simulink library "simetranss"  (R2024b)
settings: Solver=VariableStepAuto  StartTime=0.0  StopTime=10.0  RelTol=1e-3
PostLoadFcn:
  | Ts=1e-6
InitFcn:
  | Ts=1e-6
undefined symbols (not defined in the file): C, C_601, C_603, C_606, CC, Csnu, Csnubber, DiscIntNeverNeededParam, DPL, DPL1ph, FluxTable, ft2km, gcbh, h, Half, Imap2, L, L_601, L_603, L_606, Lbase, LpejoSw, Newton, R_601, R_603, R_606, Raphson, ResistanceM, Roff, Ron, RotorAngles, Rsnu, Rsnubber, Rt4, SampleTime, simetran, sps, sps_rtmsupport, StatorCurrents, T_2wind_ratio, T_Lpu, T_Lpu_pri, T_Rpu, T_Rpu_pri, T_Vpri, T_Vpri_15comp, T_Vsec, Ti, Ts_Power, Z, Zbase, Zm
libraries: fl_lib x248, ee_lib x146, nesl_utility x122, $bdroot x29, simulink x15, eeGeneralControl x2, spsStairGeneratorLib x2, artemis x1
(part 5 of 12)

== system simetranss/Lines/mate_3ph_piline ==
  Capacitor : ee_lib/Passive/Capacitor  cap_option=ee.enum.passive.capacitor.capOption.const  c=C12*len/2 F  Cvec=[1e-05, 1e-06] F  Vvec=[0, 10] V  CV_table_symmetry=ee.enum.passive.capacitor.tableSymmetry.yes  f_vec=[1, 10] kHz  DFext_vec=[.8, 1.2]  enable_C_tol=ee.enum.toleranceApplication.none  averaging_period=0 s  C_tol=5  tol_distribution=ee.enum.toleranceDistribution.uniform  nSigma=4  r=0 Ohm  g=0 1/Ohm  enable_operating_limits=ee.enum.enable.no  operating_limit_action=ee.enum.passive.reportOpLim.warn  max_working_voltage_range=[-25, 25] V  power_rating=1 W  maxTemperature=85 degC  thermalEnable=false  thermalMass=1 J/K  fault_action=simscape.enum.assert.action.none  t_fault=1 s  i_specify=off  i_priority=None  i=0 A  i_nominal_specify=off  i_nominal_value=1  i_nominal_unit=A  v_specify=off  v_priority=None  v=0 V  v_nominal_specify=off  v_nominal_value=1  v_nominal_unit=V  vc_specify=off  vc_priority=High  vc=0 V  vc_nominal_specify=off  vc_nominal_value=1  vc_nominal_unit=V  T_specify=off  T_priority=None  T=298.15 K  T_nominal_specify=off  T_nominal_value=1  T_nominal_unit=K
  Capacitor1 : ee_lib/Passive/Capacitor  cap_option=ee.enum.passive.capacitor.capOption.const  c=C23*len/2 F  Cvec=[1e-05, 1e-06] F  Vvec=[0, 10] V  CV_table_symmetry=ee.enum.passive.capacitor.tableSymmetry.yes  f_vec=[1, 10] kHz  DFext_vec=[.8, 1.2]  enable_C_tol=ee.enum.toleranceApplication.none  averaging_period=0 s  C_tol=5  tol_distribution=ee.enum.toleranceDistribution.uniform  nSigma=4  r=0 Ohm  g=0 1/Ohm  enable_operating_limits=ee.enum.enable.no  operating_limit_action=ee.enum.passive.reportOpLim.warn  max_working_voltage_range=[-25, 25] V  power_rating=1 W  maxTemperature=85 degC  thermalEnable=false  thermalMass=1 J/K  fault_action=simscape.enum.assert.action.none  t_fault=1 s  i_specify=off  i_priority=None  i=0 A  i_nominal_specify=off  i_nominal_value=1  i_nominal_unit=A  v_specify=off  v_priority=None  v=0 V  v_nominal_specify=off  v_nominal_value=1  v_nominal_unit=V  vc_specify=off  vc_priority=High  vc=0 V  vc_nominal_specify=off  vc_nominal_value=1  vc_nominal_unit=V  T_specify=off  T_priority=None  T=298.15 K  T_nominal_specify=off  T_nominal_value=1  T_nominal_unit=K
  Capacitor10 : ee_lib/Passive/Capacitor  cap_option=ee.enum.passive.capacitor.capOption.const  c=C22*len/2 F  Cvec=[1e-05, 1e-06] F  Vvec=[0, 10] V  CV_table_symmetry=ee.enum.passive.capacitor.tableSymmetry.yes  f_vec=[1, 10] kHz  DFext_vec=[.8, 1.2]  enable_C_tol=ee.enum.toleranceApplication.none  averaging_period=0 s  C_tol=5  tol_distribution=ee.enum.toleranceDistribution.uniform  nSigma=4  r=0 Ohm  g=0 1/Ohm  enable_operating_limits=ee.enum.enable.no  operating_limit_action=ee.enum.passive.reportOpLim.warn  max_working_voltage_range=[-25, 25] V  power_rating=1 W  maxTemperature=85 degC  thermalEnable=false  thermalMass=1 J/K  fault_action=simscape.enum.assert.action.none  t_fault=1 s  i_specify=off  i_priority=None  i=0 A  i_nominal_specify=off  i_nominal_value=1  i_nominal_unit=A  v_specify=off  v_priority=None  v=0 V  v_nominal_specify=off  v_nominal_value=1  v_nominal_unit=V  vc_specify=off  vc_priority=High  vc=0 V  vc_nominal_specify=off  vc_nominal_value=1  vc_nominal_unit=V  T_specify=off  T_priority=None  T=298.15 K  T_nominal_specify=off  T_nominal_value=1  T_nominal_unit=K
  Capacitor11 : ee_lib/Passive/Capacitor  cap_option=ee.enum.passive.capacitor.capOption.const  c=C33*len/2 F  Cvec=[1e-05, 1e-06] F  Vvec=[0, 10] V  CV_table_symmetry=ee.enum.passive.capacitor.tableSymmetry.yes  f_vec=[1, 10] kHz  DFext_vec=[.8, 1.2]  enable_C_tol=ee.enum.toleranceApplication.none  averaging_period=0 s  C_tol=5  tol_distribution=ee.enum.toleranceDistribution.uniform  nSigma=4  r=0 Ohm  g=0 1/Ohm  enable_operating_limits=ee.enum.enable.no  operating_limit_action=ee.enum.passive.reportOpLim.warn  max_working_voltage_range=[-25, 25] V  power_rating=1 W  maxTemperature=85 degC  thermalEnable=false  thermalMass=1 J/K  fault_action=simscape.enum.assert.action.none  t_fault=1 s  i_specify=off  i_priority=None  i=0 A  i_nominal_specify=off  i_nominal_value=1  i_nominal_unit=A  v_specify=off  v_priority=None  v=0 V  v_nominal_specify=off  v_nominal_value=1  v_nominal_unit=V  vc_specify=off  vc_priority=High  vc=0 V  vc_nominal_specify=off  vc_nominal_value=1  vc_nominal_unit=V  T_specify=off  T_priority=None  T=298.15 K  T_nominal_specify=off  T_nominal_value=1  T_nominal_unit=K
  Capacitor2 : ee_lib/Passive/Capacitor  cap_option=ee.enum.passive.capacitor.capOption.const  c=C13*len/2 F  Cvec=[1e-05, 1e-06] F  Vvec=[0, 10] V  CV_table_symmetry=ee.enum.passive.capacitor.tableSymmetry.yes  f_vec=[1, 10] kHz  DFext_vec=[.8, 1.2]  enable_C_tol=ee.enum.toleranceApplication.none  averaging_period=0 s  C_tol=5  tol_distribution=ee.enum.toleranceDistribution.uniform  nSigma=4  r=0 Ohm  g=0 1/Ohm  enable_operating_limits=ee.enum.enable.no  operating_limit_action=ee.enum.passive.reportOpLim.warn  max_working_voltage_range=[-25, 25] V  power_rating=1 W  maxTemperature=85 degC  thermalEnable=false  thermalMass=1 J/K  fault_action=simscape.enum.assert.action.none  t_fault=1 s  i_specify=off  i_priority=None  i=0 A  i_nominal_specify=off  i_nominal_value=1  i_nominal_unit=A  v_specify=off  v_priority=None  v=0 V  v_nominal_specify=off  v_nominal_value=1  v_nominal_unit=V  vc_specify=off  vc_priority=High  vc=0 V  vc_nominal_specify=off  vc_nominal_value=1  vc_nominal_unit=V  T_specify=off  T_priority=None  T=298.15 K  T_nominal_specify=off  T_nominal_value=1  T_nominal_unit=K
  Capacitor3 : ee_lib/Passive/Capacitor  cap_option=ee.enum.passive.capacitor.capOption.const  c=C23*len/2 F  Cvec=[1e-05, 1e-06] F  Vvec=[0, 10] V  CV_table_symmetry=ee.enum.passive.capacitor.tableSymmetry.yes  f_vec=[1, 10] kHz  DFext_vec=[.8, 1.2]  enable_C_tol=ee.enum.toleranceApplication.none  averaging_period=0 s  C_tol=5  tol_distribution=ee.enum.toleranceDistribution.uniform  nSigma=4  r=0 Ohm  g=0 1/Ohm  enable_operating_limits=ee.enum.enable.no  operating_limit_action=ee.enum.passive.reportOpLim.warn  max_working_voltage_range=[-25, 25] V  power_rating=1 W  maxTemperature=85 degC  thermalEnable=false  thermalMass=1 J/K  fault_action=simscape.enum.assert.action.none  t_fault=1 s  i_specify=off  i_priority=None  i=0 A  i_nominal_specify=off  i_nominal_value=1  i_nominal_unit=A  v_specify=off  v_priority=None  v=0 V  v_nominal_specify=off  v_nominal_value=1  v_nominal_unit=V  vc_specify=off  vc_priority=High  vc=0 V  vc_nominal_specify=off  vc_nominal_value=1  vc_nominal_unit=V  T_specify=off  T_priority=None  T=298.15 K  T_nominal_specify=off  T_nominal_value=1  T_nominal_unit=K
  Capacitor4 : ee_lib/Passive/Capacitor  cap_option=ee.enum.passive.capacitor.capOption.const  c=C12*len/2 F  Cvec=[1e-05, 1e-06] F  Vvec=[0, 10] V  CV_table_symmetry=ee.enum.passive.capacitor.tableSymmetry.yes  f_vec=[1, 10] kHz  DFext_vec=[.8, 1.2]  enable_C_tol=ee.enum.toleranceApplication.none  averaging_period=0 s  C_tol=5  tol_distribution=ee.enum.toleranceDistribution.uniform  nSigma=4  r=0 Ohm  g=0 1/Ohm  enable_operating_limits=ee.enum.enable.no  operating_limit_action=ee.enum.passive.reportOpLim.warn  max_working_voltage_range=[-25, 25] V  power_rating=1 W  maxTemperature=85 degC  thermalEnable=false  thermalMass=1 J/K  fault_action=simscape.enum.assert.action.none  t_fault=1 s  i_specify=off  i_priority=None  i=0 A  i_nominal_specify=off  i_nominal_value=1  i_nominal_unit=A  v_specify=off  v_priority=None  v=0 V  v_nominal_specify=off  v_nominal_value=1  v_nominal_unit=V  vc_specify=off  vc_priority=High  vc=0 V  vc_nominal_specify=off  vc_nominal_value=1  vc_nominal_unit=V  T_specify=off  T_priority=None  T=298.15 K  T_nominal_specify=off  T_nominal_value=1  T_nominal_unit=K
  Capacitor5 : ee_lib/Passive/Capacitor  cap_option=ee.enum.passive.capacitor.capOption.const  c=C13*len/2 F  Cvec=[1e-05, 1e-06] F  Vvec=[0, 10] V  CV_table_symmetry=ee.enum.passive.capacitor.tableSymmetry.yes  f_vec=[1, 10] kHz  DFext_vec=[.8, 1.2]  enable_C_tol=ee.enum.toleranceApplication.none  averaging_period=0 s  C_tol=5  tol_distribution=ee.enum.toleranceDistribution.uniform  nSigma=4  r=0 Ohm  g=0 1/Ohm  enable_operating_limits=ee.enum.enable.no  operating_limit_action=ee.enum.passive.reportOpLim.warn  max_working_voltage_range=[-25, 25] V  power_rating=1 W  maxTemperature=85 degC  thermalEnable=false  thermalMass=1 J/K  fault_action=simscape.enum.assert.action.none  t_fault=1 s  i_specify=off  i_priority=None  i=0 A  i_nominal_specify=off  i_nominal_value=1  i_nominal_unit=A  v_specify=off  v_priority=None  v=0 V  v_nominal_specify=off  v_nominal_value=1  v_nominal_unit=V  vc_specify=off  vc_priority=High  vc=0 V  vc_nominal_specify=off  vc_nominal_value=1  vc_nominal_unit=V  T_specify=off  T_priority=None  T=298.15 K  T_nominal_specify=off  T_nominal_value=1  T_nominal_unit=K
  Capacitor6 : ee_lib/Passive/Capacitor  cap_option=ee.enum.passive.capacitor.capOption.const  c=C11*len/2 F  Cvec=[1e-05, 1e-06] F  Vvec=[0, 10] V  CV_table_symmetry=ee.enum.passive.capacitor.tableSymmetry.yes  f_vec=[1, 10] kHz  DFext_vec=[.8, 1.2]  enable_C_tol=ee.enum.toleranceApplication.none  averaging_period=0 s  C_tol=5  tol_distribution=ee.enum.toleranceDistribution.uniform  nSigma=4  r=0 Ohm  g=0 1/Ohm  enable_operating_limits=ee.enum.enable.no  operating_limit_action=ee.enum.passive.reportOpLim.warn  max_working_voltage_range=[-25, 25] V  power_rating=1 W  maxTemperature=85 degC  thermalEnable=false  thermalMass=1 J/K  fault_action=simscape.enum.assert.action.none  t_fault=1 s  i_specify=off  i_priority=None  i=0 A  i_nominal_specify=off  i_nominal_value=1  i_nominal_unit=A  v_specify=off  v_priority=None  v=0 V  v_nominal_specify=off  v_nominal_value=1  v_nominal_unit=V  vc_specify=off  vc_priority=High  vc=0 V  vc_nominal_specify=off  vc_nominal_value=1  vc_nominal_unit=V  T_specify=off  T_priority=None  T=298.15 K  T_nominal_specify=off  T_nominal_value=1  T_nominal_unit=K
  Capacitor7 : ee_lib/Passive/Capacitor  cap_option=ee.enum.passive.capacitor.capOption.const  c=C22*len/2 F  Cvec=[1e-05, 1e-06] F  Vvec=[0, 10] V  CV_table_symmetry=ee.enum.passive.capacitor.tableSymmetry.yes  f_vec=[1, 10] kHz  DFext_vec=[.8, 1.2]  enable_C_tol=ee.enum.toleranceApplication.none  averaging_period=0 s  C_tol=5  tol_distribution=ee.enum.toleranceDistribution.uniform  nSigma=4  r=0 Ohm  g=0 1/Ohm  enable_operating_limits=ee.enum.enable.no  operating_limit_action=ee.enum.passive.reportOpLim.warn  max_working_voltage_range=[-25, 25] V  power_rating=1 W  maxTemperature=85 degC  thermalEnable=false  thermalMass=1 J/K  fault_action=simscape.enum.assert.action.none  t_fault=1 s  i_specify=off  i_priority=None  i=0 A  i_nominal_specify=off  i_nominal_value=1  i_nominal_unit=A  v_specify=off  v_priority=None  v=0 V  v_nominal_specify=off  v_nominal_value=1  v_nominal_unit=V  vc_specify=off  vc_priority=High  vc=0 V  vc_nominal_specify=off  vc_nominal_value=1  vc_nominal_unit=V  T_specify=off  T_priority=None  T=298.15 K  T_nominal_specify=off  T_nominal_value=1  T_nominal_unit=K
  Capacitor8 : ee_lib/Passive/Capacitor  cap_option=ee.enum.passive.capacitor.capOption.const  c=C33*len/2 F  Cvec=[1e-05, 1e-06] F  Vvec=[0, 10] V  CV_table_symmetry=ee.enum.passive.capacitor.tableSymmetry.yes  f_vec=[1, 10] kHz  DFext_vec=[.8, 1.2]  enable_C_tol=ee.enum.toleranceApplication.none  averaging_period=0 s  C_tol=5  tol_distribution=ee.enum.toleranceDistribution.uniform  nSigma=4  r=0 Ohm  g=0 1/Ohm  enable_operating_limits=ee.enum.enable.no  operating_limit_action=ee.enum.passive.reportOpLim.warn  max_working_voltage_range=[-25, 25] V  power_rating=1 W  maxTemperature=85 degC  thermalEnable=false  thermalMass=1 J/K  fault_action=simscape.enum.assert.action.none  t_fault=1 s  i_specify=off  i_priority=None  i=0 A  i_nominal_specify=off  i_nominal_value=1  i_nominal_unit=A  v_specify=off  v_priority=None  v=0 V  v_nominal_specify=off  v_nominal_value=1  v_nominal_unit=V  vc_specify=off  vc_priority=High  vc=0 V  vc_nominal_specify=off  vc_nominal_value=1  vc_nominal_unit=V  T_specify=off  T_priority=None  T=298.15 K  T_nominal_specify=off  T_nominal_value=1  T_nominal_unit=K
  Capacitor9 : ee_lib/Passive/Capacitor  cap_option=ee.enum.passive.capacitor.capOption.const  c=C11*len/2 F  Cvec=[1e-05, 1e-06] F  Vvec=[0, 10] V  CV_table_symmetry=ee.enum.passive.capacitor.tableSymmetry.yes  f_vec=[1, 10] kHz  DFext_vec=[.8, 1.2]  enable_C_tol=ee.enum.toleranceApplication.none  averaging_period=0 s  C_tol=5  tol_distribution=ee.enum.toleranceDistribution.uniform  nSigma=4  r=0 Ohm  g=0 1/Ohm  enable_operating_limits=ee.enum.enable.no  operating_limit_action=ee.enum.passive.reportOpLim.warn  max_working_voltage_range=[-25, 25] V  power_rating=1 W  maxTemperature=85 degC  thermalEnable=false  thermalMass=1 J/K  fault_action=simscape.enum.assert.action.none  t_fault=1 s  i_specify=off  i_priority=None  i=0 A  i_nominal_specify=off  i_nominal_value=1  i_nominal_unit=A  v_specify=off  v_priority=None  v=0 V  v_nominal_specify=off  v_nominal_value=1  v_nominal_unit=V  vc_specify=off  vc_priority=High  vc=0 V  vc_nominal_specify=off  vc_nominal_value=1  vc_nominal_unit=V  T_specify=off  T_priority=None  T=298.15 K  T_nominal_specify=off  T_nominal_value=1  T_nominal_unit=K
  Coupled Lines (Three-Phase) : ee_lib/Passive/Lines/Coupled Lines (Three-Phase)  prm=2  La=LL(1,1)*len H  Lb=LL(2,2)*len H  Lc=LL(3,3)*len H  L=1e-3 H  Lmab=LL(1,2)*len H  Lmac=LL(1,3)*len H  Lmbc=LL(2,3)*len H  Lm=3e-4 H  Ra=RR(1,1)*len Ohm  Rb=RR(2,2)*len Ohm  Rc=RR(3,3)*len Ohm  R=0.001 Ohm  Rm=(RR(1,2)+RR(1,3)+RR(2,3))/3*len Ohm  Ga=1e-9 1/Ohm  Gb=1e-9 1/Ohm  Gc=1e-9 1/Ohm  G=1e-9 1/Ohm  I_L_specify=off  I_L_priority=High  I_L=[0, 0, 0] A  I_L_nominal_specify=off  I_L_nominal_value=1  I_L_nominal_unit=A  i_La_specify=off  i_La_priority=High  i_La=0 A  i_La_nominal_specify=off  i_La_nominal_value=1  i_La_nominal_unit=A  i_Lb_specify=off  i_Lb_priority=High  i_Lb=0 A  i_Lb_nominal_specify=off  i_Lb_nominal_value=1  i_Lb_nominal_unit=A  i_Lc_specify=off  i_Lc_priority=High  i_Lc=0 A  i_Lc_nominal_specify=off  i_Lc_nominal_value=1  i_Lc_nominal_unit=A
      settings: InternalSimscapePortConfiguration="{\"Bottom\":[],\"Left\":[{\"id\":\"a1\",\"label\":\"a1\",\"type\":\"foundation.electrical.electrical\"},{\"id\":\"b1\",\"label\":\"b1\",\"type\":\"foundation.electrical.electrical\"},{\"id\":\"c1\",\"label\":\"c1\",\"type\":\"foundation.electrical.electrical\"}],\"Right\":[{\"id\":\"a2\",\"label\":\"a2\",\"type\":\"foundation.electrical.electrical\"},{\"id\":\"b2\",\"label\":\"b2\",\"type\":\"foundation.electrical.electrical\"},{\"id\":\"c2\",\"label\":\"c2\",\"type\":\"foundation.electrical.electrical\"}],\"Top\":[]}"
  Electrical Reference : fl_lib/Electrical/Electrical Elements/Electrical Reference
  Electrical Reference1 : fl_lib/Electrical/Electrical Elements/Electrical Reference
  Phase Splitter1 : ee_lib/Connectors & References/Phase Splitter
  Phase Splitter2 : ee_lib/Connectors & References/Phase Splitter
  abc : PMIOPort  Side=Left
  .abc : PMIOPort  Port=2  Side=Right
  connections:
  .abc/RConn1 -- Phase Splitter1/LConn1
  Phase Splitter2/LConn1 -- abc/RConn1
  Phase Splitter2/RConn3 -- Capacitor1/RConn1 -- Coupled Lines (Three-Phase)/LConn3 -- Capacitor8/LConn1 -- Capacitor2/RConn1
  Coupled Lines (Three-Phase)/RConn3 -- Capacitor3/LConn1 -- Capacitor5/LConn1 -- Phase Splitter1/RConn3 -- Capacitor11/LConn1
  Phase Splitter2/RConn1 -- Capacitor6/LConn1 -- Coupled Lines (Three-Phase)/LConn1 -- Capacitor/LConn1 -- Capacitor2/LConn1
  Phase Splitter1/RConn1 -- Capacitor4/RConn1 -- Capacitor9/LConn1 -- Coupled Lines (Three-Phase)/RConn1 -- Capacitor5/RConn1
  Capacitor7/RConn1 -- Capacitor8/RConn1 -- Capacitor6/RConn1 -- Electrical Reference/LConn1
  Coupled Lines (Three-Phase)/LConn2 -- Capacitor/RConn1 -- Capacitor1/LConn1 -- Phase Splitter2/RConn2 -- Capacitor7/LConn1
  Phase Splitter1/RConn2 -- Capacitor4/LConn1 -- Coupled Lines (Three-Phase)/RConn2 -- Capacitor10/LConn1 -- Capacitor3/RConn1
  Electrical Reference1/LConn1 -- Capacitor9/RConn1 -- Capacitor11/RConn1 -- Capacitor10/RConn1

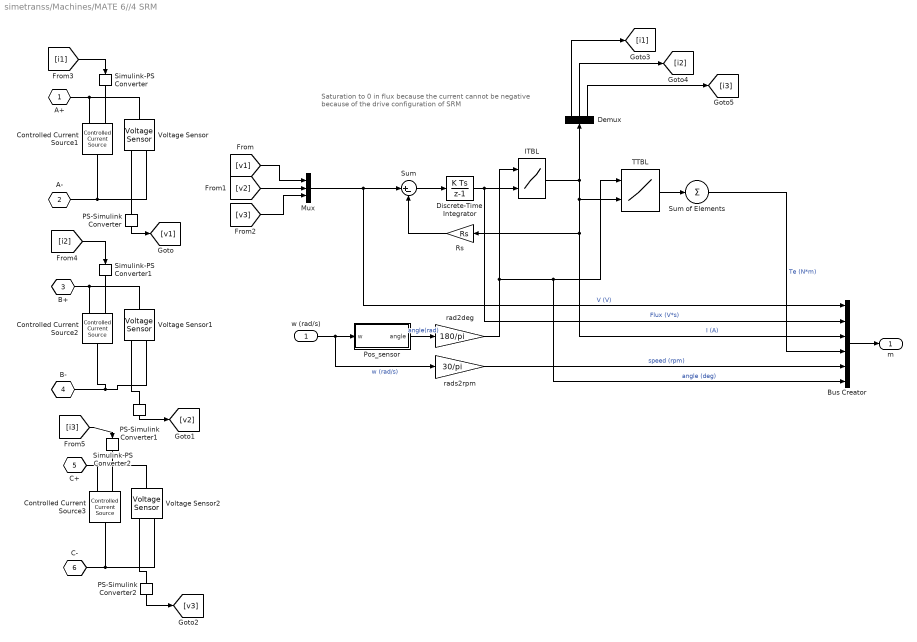
== system simetranss/Machines/MATE 6//4 SRM ==
  note: Saturation to 0 in flux because the current cannot be negative
      | because of the drive configuration of SRM
  w (rad/s) : Inport
  Bus Creator : BusCreator  Inputs=6
  Controlled Current Source1 : fl_lib/Electrical/Electrical Sources/Controlled Current Source
  Controlled Current Source2 : fl_lib/Electrical/Electrical Sources/Controlled Current Source
  Controlled Current Source3 : fl_lib/Electrical/Electrical Sources/Controlled Current Source
  Demux : Demux  Outputs=3
  Discrete-Time Integrator : DiscreteIntegrator  SampleTime=Ts  LimitOutput=on  LowerSaturationLimit=0  ICPrevOutput=DiscIntNeverNeededParam  ICPrevScaledInput=DiscIntNeverNeededParam
  ITBL : Lookup2D  RowIndex=theta2  ColumnIndex=all_flux_value  Table=Imap2'  InputSameDT=off
  Mux : Mux  Inputs=3
  PS-Simulink Converter : nesl_utility/PS-Simulink Converter  PhysicalDomain=network_engine_domain  SubClassName=ps_output  LeftPortType=input  RightPortType=output  PseudoPeriodic=off  Frequencies=[]  VectorFormat=inherit  Unit=inherit  AffineConversion=off
  PS-Simulink Converter1 : nesl_utility/PS-Simulink Converter  PhysicalDomain=network_engine_domain  SubClassName=ps_output  LeftPortType=input  RightPortType=output  PseudoPeriodic=off  Frequencies=[]  VectorFormat=inherit  Unit=inherit  AffineConversion=off
  PS-Simulink Converter2 : nesl_utility/PS-Simulink Converter  PhysicalDomain=network_engine_domain  SubClassName=ps_output  LeftPortType=input  RightPortType=output  PseudoPeriodic=off  Frequencies=[]  VectorFormat=inherit  Unit=inherit  AffineConversion=off
  Pos_sensor : Subsystem
  Rs : Gain  Gain=Rs  SaturateOnIntegerOverflow=on  OutDataTypeStr=Inherit: Same as input  ParamDataTypeStr=Inherit: Same as input
  Simulink-PS Converter : nesl_utility/Simulink-PS Converter  PhysicalDomain=network_engine_domain  SubClassName=ps_input  LeftPortType=input  RightPortType=output  PseudoPeriodic=off  Frequencies=[]  NoiseDistribution=none  NoiseParameters=[]  Unit=1  AffineConversion=off  FilteringAndDerivatives=provide  SimscapeFilterOrder=1  InputFilterTimeConstant=0.001  UdotUserProvided=0
  Simulink-PS Converter1 : nesl_utility/Simulink-PS Converter  PhysicalDomain=network_engine_domain  SubClassName=ps_input  LeftPortType=input  RightPortType=output  PseudoPeriodic=off  Frequencies=[]  NoiseDistribution=none  NoiseParameters=[]  Unit=1  AffineConversion=off  FilteringAndDerivatives=provide  SimscapeFilterOrder=1  InputFilterTimeConstant=0.001  UdotUserProvided=0
  Simulink-PS Converter2 : nesl_utility/Simulink-PS Converter  PhysicalDomain=network_engine_domain  SubClassName=ps_input  LeftPortType=input  RightPortType=output  PseudoPeriodic=off  Frequencies=[]  NoiseDistribution=none  NoiseParameters=[]  Unit=1  AffineConversion=off  FilteringAndDerivatives=provide  SimscapeFilterOrder=1  InputFilterTimeConstant=0.001  UdotUserProvided=0
  Sum : Sum  Inputs=|+-  SaturateOnIntegerOverflow=on
  Sum of Elements : Sum  Inputs=1  SampleTime=Ts
  TTBL : Lookup2D  RowIndex=theta2  ColumnIndex=Icoil2  Table=Temap'  InputSameDT=off
  Voltage Sensor : fl_lib/Electrical/Electrical Sensors/Voltage Sensor
  Voltage Sensor1 : fl_lib/Electrical/Electrical Sensors/Voltage Sensor
  Voltage Sensor2 : fl_lib/Electrical/Electrical Sensors/Voltage Sensor
  rad2deg : Gain  Gain=180/pi  SaturateOnIntegerOverflow=on  OutDataTypeStr=Inherit: Same as input  ParamDataTypeStr=Inherit: Same as input
  rads2rpm : Gain  Gain=30/pi  SaturateOnIntegerOverflow=on  OutDataTypeStr=Inherit: Same as input  ParamDataTypeStr=Inherit: Same as input
  A+ : PMIOPort  Side=Left
  A- : PMIOPort  Port=2  Side=Left
  B+ : PMIOPort  Port=3  Side=Left
  B- : PMIOPort  Port=4  Side=Left
  C+ : PMIOPort  Port=5  Side=Left
  C- : PMIOPort  Port=6  Side=Left
  m : Outport  VectorParamsAs1DForOutWhenUnconnected=off
  wires:
  [i3] -> Simulink-PS Converter2/1
  [i2] -> Simulink-PS Converter1/1
  [i1] -> Simulink-PS Converter/1
  Demux/3 -> [i3]
  Demux/2 -> [i2]
  Demux/1 -> [i1]
  [v3] -> Mux/3
  [v1] -> Mux/1
  [v2] -> Mux/2
  PS-Simulink Converter2/1 -> [v3]
  PS-Simulink Converter1/1 -> [v2]
  PS-Simulink Converter/1 -> [v1]
  rads2rpm/1 -> Bus Creator/5  "speed (rpm)"
  rad2deg/1 -> ITBL/1, Bus Creator/6, TTBL/1  "angle (deg)"
  Pos_sensor/1(angle) -> rad2deg/1  "angle(rad)"
  Mux/1 -> Bus Creator/1, Sum/1  "V (V)"
  Rs/1 -> Sum/2
  Sum of Elements/1 -> Bus Creator/4  "Te (N*m)"
  Bus Creator/1 -> m/1
  w (rad/s)/1 -> Pos_sensor/1(w), rads2rpm/1  "w (rad/s)"
  ITBL/1 -> Demux/1, TTBL/2, Rs/1, Bus Creator/3  "I (A)"
  Sum/1 -> Discrete-Time Integrator/1
  Discrete-Time Integrator/1 -> ITBL/2, Bus Creator/2  "Flux (V*s)"
  TTBL/1 -> Sum of Elements/1
  connections:
  PS-Simulink Converter2/LConn1 -- Voltage Sensor2/RConn1
  Simulink-PS Converter2/RConn1 -- Controlled Current Source3/RConn1
  Controlled Current Source3/RConn2 -- Voltage Sensor2/LConn1 -- C+/RConn1
  Controlled Current Source3/LConn1 -- C-/RConn1 -- Voltage Sensor2/RConn2
  Simulink-PS Converter1/RConn1 -- Controlled Current Source2/RConn1
  PS-Simulink Converter1/LConn1 -- Voltage Sensor1/RConn1
  Controlled Current Source2/RConn2 -- B+/RConn1 -- Voltage Sensor1/LConn1
  Voltage Sensor1/RConn2 -- B-/RConn1 -- Controlled Current Source2/LConn1
  PS-Simulink Converter/LConn1 -- Voltage Sensor/RConn1
  Simulink-PS Converter/RConn1 -- Controlled Current Source1/RConn1
  Voltage Sensor/LConn1 -- A+/RConn1 -- Controlled Current Source1/RConn2
  Controlled Current Source1/LConn1 -- A-/RConn1 -- Voltage Sensor/RConn2

== system simetranss/Machines/MATE Brushless DC Motor (ALT1) ==
  "   w_mec" : Inport
  Bias : Bias  Bias=[0 -2*pi/3 2*pi/3]  SaturateOnIntegerOverflow=off
  Bus Creator : BusCreator  Inputs=5
  Controlled Voltage Source (Three-Phase) : ee_lib/Sources/Controlled Voltage Source (Three-Phase)  input_option=ee.enum.inputType.instantaneous  FRated=60 Hz
      settings: InternalSimscapePortConfiguration="{\"Bottom\":[],\"Left\":[{\"id\":\"S\",\"label\":\"S\",\"type\":\"input\"},{\"id\":\"n\",\"label\":\"n\",\"type\":\"foundation.electrical.electrical\"}],\"Right\":[{\"id\":\"N\",\"label\":\"~\",\"type\":\"foundation.electrical.three_phase\"}],\"Top\":[]}"
  Coupled Lines (Three-Phase) : ee_lib/Passive/Lines/Coupled Lines (Three-Phase)  prm=1  La=1e-3 H  Lb=1e-3 H  Lc=1e-3 H  L=2*Ld H  Lmab=3e-4 H  Lmac=3e-4 H  Lmbc=3e-4 H  Lm=Ld H  Ra=0.001 Ohm  Rb=0.001 Ohm  Rc=0.001 Ohm  R=Rs Ohm  Rm=0 Ohm  Ga=1e-9 1/Ohm  Gb=1e-9 1/Ohm  Gc=1e-9 1/Ohm  G=1e-9 1/Ohm  I_L_specify=off  I_L_priority=High  I_L=[0, 0, 0] A  I_L_nominal_specify=off  I_L_nominal_value=1  I_L_nominal_unit=A  i_La_specify=off  i_La_priority=High  i_La=0 A  i_La_nominal_specify=off  i_La_nominal_value=1  i_La_nominal_unit=A  i_Lb_specify=off  i_Lb_priority=High  i_Lb=0 A  i_Lb_nominal_specify=off  i_Lb_nominal_value=1  i_Lb_nominal_unit=A  i_Lc_specify=off  i_Lc_priority=High  i_Lc=0 A  i_Lc_nominal_specify=off  i_Lc_nominal_value=1  i_Lc_nominal_unit=A
      settings: InternalSimscapePortConfiguration="{\"Bottom\":[],\"Left\":[{\"id\":\"N1\",\"label\":\"~1\",\"type\":\"foundation.electrical.three_phase\"}],\"Right\":[{\"id\":\"N2\",\"label\":\"~2\",\"type\":\"foundation.electrical.three_phase\"}],\"Top\":[]}"
  Current Sensor (Three-Phase) : ee_lib/Sensors & Transducers/Current Sensor (Three-Phase)
  Discrete-Time Integrator : DiscreteIntegrator  InitialCondition=pp*AngInit/180*pi  SampleTime=Ts  ICPrevOutput=DiscIntNeverNeededParam  ICPrevScaledInput=DiscIntNeverNeededParam
  Gain1 : Gain  Gain=1/pp
  Gain3 : Gain  Gain=pp  SaturateOnIntegerOverflow=on  OutDataTypeStr=Inherit: Same as input  ParamDataTypeStr=Inherit: Same as input
  Gain4 : Gain  Gain=-Mf
  PS-Simulink Converter4 : nesl_utility/PS-Simulink Converter  PhysicalDomain=network_engine_domain  SubClassName=ps_output  LeftPortType=input  RightPortType=output  PseudoPeriodic=off  Frequencies=[]  VectorFormat=inherit  Unit=inherit  AffineConversion=off
  Product6 : Product  RndMeth=Zero
  Product8 : Product  SaturateOnIntegerOverflow=on  OutDataTypeStr=Inherit: Same as first input
  Signal Specification : SignalSpecification  Dimensions=3
  Simulink-PS Converter3 : nesl_utility/Simulink-PS Converter  PhysicalDomain=network_engine_domain  SubClassName=ps_input  LeftPortType=input  RightPortType=output  PseudoPeriodic=off  Frequencies=[]  NoiseDistribution=none  NoiseParameters=[]  Unit=1  AffineConversion=off  FilteringAndDerivatives=provide  SimscapeFilterOrder=1  InputFilterTimeConstant=0.001  UdotUserProvided=0
  Sum2 : Sum  Inputs=+  SaturateOnIntegerOverflow=on
  Trigonometric Function1 : Trigonometry
  pole pair1 : Gain  Gain=pp
  "   abc" : PMIOPort  Side=Left
  meas : Outport  VectorParamsAs1DForOutWhenUnconnected=off
  wires:
  [Te] -> Bus Creator/3  "Electric torque (Nm)"
  Bus Creator/1 -> meas/1
  "   w_mec"/1 -> pole pair1/1, [W_m]
  pole pair1/1 -> Discrete-Time Integrator/1, [w_e]  "w_elect"
  Discrete-Time Integrator/1 -> [theta_e], Gain1/1  "theta_elect (rad)"
  [iabc_bldc] -> Signal Specification/1  "Iabc(A)"
  [backemf] -> Bus Creator/2  "Back-EMF (V)"
  Gain1/1 -> [Theta_m]
  [W_m] -> Bus Creator/5  "mec speed (rad_s)"
  [Theta_m] -> Bus Creator/4  "mec angle (rad)"
  [theta_e] -> Bias/1
  Bias/1 -> Trigonometric Function1/1
  [w_e] -> Product6/2
  Trigonometric Function1/1 -> Gain4/1
  Product6/1 -> Simulink-PS Converter3/1, [backemf]  "BackEMF on q axis"
  Gain3/1 -> [Te]
  Product8/1 -> Sum2/1
  [iabc_bldc] -> Product8/2
  [X] -> Product8/1
  Sum2/1 -> Gain3/1
  PS-Simulink Converter4/1 -> [iabc_bldc]
  Gain4/1 -> Product6/1, [X]
  Signal Specification/1 -> Bus Creator/1  "Iabc(A)"
  connections:
  Controlled Voltage Source (Three-Phase)/RConn1 -- Coupled Lines (Three-Phase)/RConn1
  Simulink-PS Converter3/RConn1 -- Controlled Voltage Source (Three-Phase)/LConn1
  PS-Simulink Converter4/LConn1 -- Current Sensor (Three-Phase)/RConn1
  Current Sensor (Three-Phase)/LConn1 -- "   abc"/RConn1
  Coupled Lines (Three-Phase)/LConn1 -- Current Sensor (Three-Phase)/RConn2

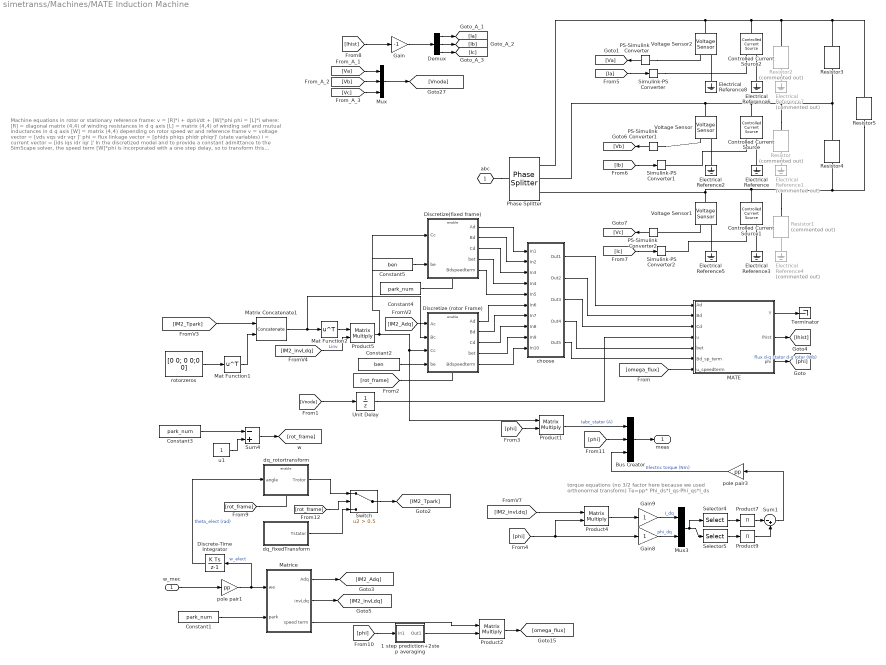
== system simetranss/Machines/MATE Induction Machine ==
  note: Machine equations in rotor or stationary reference frame:
      |
      |   v = [R]*i + dphi/dt + [W]*phi
      | phi = [L]*i
      |
      | where:
      | [R] = diagonal matrix (4,4) of winding resistances in d q axis
      | [L] = matrix (4,4) of winding self and mutual inductances in d q axis
      | [W] = matrix (4,4) depending on rotor speed wr and reference frame
      |
      |   v = voltage vector      = [vds   vqs   vdr   vqr  ]'
      | phi = flux linkage vector = [phids phiqs phidr phiqr]' (state variables)
      |   i = current vector      = [ids   iqs   idr   iqr  ]'
      |
      | In the discretized model and to provide a constant admittance to the SimScape solver, the speed term [W]*phi is incorporated with a one step delay, so to transform this component into an input to the state equations
  note: torque equations
      | (no 3/2 factor here because we used orthonormal transform)
      | Te=pp* Phi_ds*I_qs-Phi_qs*I_ds
  "   w_mec" : Inport
  1 step prediction+2step averaging : Subsystem
  Bus Creator : BusCreator  Inputs=3
  Constant1 : Constant  Value=park_num
  Constant2 : Constant  Value=ben
  Constant3 : Constant  Value=park_num
  Constant4 : Constant  Value=park_num
  Constant5 : Constant  Value=ben
  Controlled Current Source : fl_lib/Electrical/Electrical Sources/Controlled Current Source
  Controlled Current Source1 : fl_lib/Electrical/Electrical Sources/Controlled Current Source
  Controlled Current Source2 : fl_lib/Electrical/Electrical Sources/Controlled Current Source
  Demux : Demux  Outputs=3
      settings: DisplayOption=none
  Discrete-Time Integrator : DiscreteIntegrator  SampleTime=Ts  ICPrevOutput=DiscIntNeverNeededParam  ICPrevScaledInput=DiscIntNeverNeededParam
  Discretize (rotor Frame) : Subsystem
  Discretize(fixed frame) : Subsystem
  Electrical Reference{,2..3,5..6,8} (6 alike) : fl_lib/Electrical/Electrical Elements/Electrical Reference
  Electrical Reference1 : fl_lib/Electrical/Electrical Elements/Electrical Reference  Commented=on
  Electrical Reference4 : fl_lib/Electrical/Electrical Elements/Electrical Reference  Commented=on
  Electrical Reference7 : fl_lib/Electrical/Electrical Elements/Electrical Reference  Commented=on
  Gain : Gain  Gain=-1
  Gain8 : Gain
  Gain9 : Gain
  MATE : Subsystem
  Mat Function1 : Math  Operator=transpose  SignedPower=on
  Mat Function2 : Math  Operator=transpose  SignedPower=on
  Matrice : Subsystem
  Matrix Concatenate1 : Concatenate  Mode=Multidimensional array
  Mux : Mux  Inputs=3
  Mux3 : Mux  Inputs=2
  PS-Simulink Converter : nesl_utility/PS-Simulink Converter  PhysicalDomain=network_engine_domain  SubClassName=ps_output  LeftPortType=input  RightPortType=output  PseudoPeriodic=off  Frequencies=[]  VectorFormat=inherit  Unit=inherit  AffineConversion=off
  PS-Simulink Converter1 : nesl_utility/PS-Simulink Converter  PhysicalDomain=network_engine_domain  SubClassName=ps_output  LeftPortType=input  RightPortType=output  PseudoPeriodic=off  Frequencies=[]  VectorFormat=inherit  Unit=inherit  AffineConversion=off
  PS-Simulink Converter2 : nesl_utility/PS-Simulink Converter  PhysicalDomain=network_engine_domain  SubClassName=ps_output  LeftPortType=input  RightPortType=output  PseudoPeriodic=off  Frequencies=[]  VectorFormat=inherit  Unit=inherit  AffineConversion=off
  Phase Splitter : ee_lib/Connectors & References/Phase Splitter
  Product{1..2,4..5} (4 alike) : Product  Multiplication=Matrix(*)  SaturateOnIntegerOverflow=on  OutDataTypeStr=Inherit: Same as first input
  Product7 : Product  Inputs=1  InputSameDT=on  SaturateOnIntegerOverflow=on  OutDataTypeStr=Inherit: Same as first input
  Product9 : Product  Inputs=1  InputSameDT=on  SaturateOnIntegerOverflow=on  OutDataTypeStr=Inherit: Same as first input
  Resistor : fl_lib/Electrical/Electrical Elements/Resistor  Commented=on  R=ResistanceM(2,2) Ohm  i_specify=off  i_priority=None  i=0 A  i_nominal_specify=off  i_nominal_value=1  i_nominal_unit=A  v_specify=off  v_priority=None  v=0 V  v_nominal_specify=off  v_nominal_value=1  v_nominal_unit=V
  Resistor1 : fl_lib/Electrical/Electrical Elements/Resistor  Commented=on  R=ResistanceM(3,3) Ohm  i_specify=off  i_priority=None  i=0 A  i_nominal_specify=off  i_nominal_value=1  i_nominal_unit=A  v_specify=off  v_priority=None  v=0 V  v_nominal_specify=off  v_nominal_value=1  v_nominal_unit=V
  Resistor2 : fl_lib/Electrical/Electrical Elements/Resistor  Commented=on  R=ResistanceM(1,1) Ohm  i_specify=off  i_priority=None  i=0 A  i_nominal_specify=off  i_nominal_value=1  i_nominal_unit=A  v_specify=off  v_priority=None  v=0 V  v_nominal_specify=off  v_nominal_value=1  v_nominal_unit=V
  Resistor3 : fl_lib/Electrical/Electrical Elements/Resistor  R=ResistanceM(1,2) Ohm  i_specify=off  i_priority=None  i=0 A  i_nominal_specify=off  i_nominal_value=1  i_nominal_unit=A  v_specify=off  v_priority=None  v=0 V  v_nominal_specify=off  v_nominal_value=1  v_nominal_unit=V
  Resistor4 : fl_lib/Electrical/Electrical Elements/Resistor  R=ResistanceM(2,3) Ohm  i_specify=off  i_priority=None  i=0 A  i_nominal_specify=off  i_nominal_value=1  i_nominal_unit=A  v_specify=off  v_priority=None  v=0 V  v_nominal_specify=off  v_nominal_value=1  v_nominal_unit=V
  Resistor5 : fl_lib/Electrical/Electrical Elements/Resistor  R=ResistanceM(1,3) Ohm  i_specify=off  i_priority=None  i=0 A  i_nominal_specify=off  i_nominal_value=1  i_nominal_unit=A  v_specify=off  v_priority=None  v=0 V  v_nominal_specify=off  v_nominal_value=1  v_nominal_unit=V
  Selector4 : Selector  InputPortWidth=8  IndexOptions=Index vector (dialog)  Indices=[1 6]  OutputSizes=1
  Selector5 : Selector  InputPortWidth=8  IndexOptions=Index vector (dialog)  Indices=[2 5]  OutputSizes=1
  Simulink-PS Converter : nesl_utility/Simulink-PS Converter  PhysicalDomain=network_engine_domain  SubClassName=ps_input  LeftPortType=input  RightPortType=output  PseudoPeriodic=off  Frequencies=[]  NoiseDistribution=none  NoiseParameters=[]  Unit=1  AffineConversion=off  FilteringAndDerivatives=provide  SimscapeFilterOrder=1  InputFilterTimeConstant=0.001  UdotUserProvided=0
  Simulink-PS Converter1 : nesl_utility/Simulink-PS Converter  PhysicalDomain=network_engine_domain  SubClassName=ps_input  LeftPortType=input  RightPortType=output  PseudoPeriodic=off  Frequencies=[]  NoiseDistribution=none  NoiseParameters=[]  Unit=1  AffineConversion=off  FilteringAndDerivatives=provide  SimscapeFilterOrder=1  InputFilterTimeConstant=0.001  UdotUserProvided=0
  Simulink-PS Converter2 : nesl_utility/Simulink-PS Converter  PhysicalDomain=network_engine_domain  SubClassName=ps_input  LeftPortType=input  RightPortType=output  PseudoPeriodic=off  Frequencies=[]  NoiseDistribution=none  NoiseParameters=[]  Unit=1  AffineConversion=off  FilteringAndDerivatives=provide  SimscapeFilterOrder=1  InputFilterTimeConstant=0.001  UdotUserProvided=0
  Sum1 : Sum  Inputs=|-+  InputSameDT=on  SaturateOnIntegerOverflow=on  OutDataTypeStr=Inherit: Same as first input
  Sum4 : Sum  Inputs=-+  SaturateOnIntegerOverflow=on
  Switch : Switch  Criteria=u2 > Threshold  Threshold=0.5  SaturateOnIntegerOverflow=off  InputSameDT=off
  Terminator : Terminator
  Unit Delay : UnitDelay  SampleTime=Ts  HasFrameUpgradeWarning=on
  Voltage Sensor : fl_lib/Electrical/Electrical Sensors/Voltage Sensor
  Voltage Sensor1 : fl_lib/Electrical/Electrical Sensors/Voltage Sensor
  Voltage Sensor2 : fl_lib/Electrical/Electrical Sensors/Voltage Sensor
  choose : Subsystem
  dq_fixedTransform : Subsystem
  dq_rotortransform : Subsystem
  pole pair1 : Gain  Gain=pp
  pole pair3 : Gain  Gain=pp
  rotorzeros : Constant  Value=[0 0; 0 0;0 0]
  u1 : Constant
  "   abc" : PMIOPort  Side=Left
  meas : Outport  VectorParamsAs1DForOutWhenUnconnected=off
  wires:
  dq_fixedTransform/1(Tstator) -> Switch/3
  [rot_frame] -> dq_rotortransform/Enable
  [rot_frame] -> Switch/2
  choose/5(Out5) -> MATE/6(Bd_sp_term)
  choose/4(Out4) -> MATE/5(bet)
  choose/3(Out3) -> MATE/3(Cd)
  choose/2(Out2) -> MATE/2(Bd)
  choose/1(Out1) -> MATE/1(Ad)
  Discretize (rotor Frame)/5(Bdspeedterm) -> choose/10(In10)
  Discretize (rotor Frame)/4(bet) -> choose/9(In9)
  Discretize (rotor Frame)/3(Cd) -> choose/8(In8)
  Discretize (rotor Frame)/2(Bd) -> choose/7(In7)
  Discretize (rotor Frame)/1(Ad) -> choose/6(In6)
  Discretize(fixed frame)/5(Bdspeedterm) -> choose/5(In5)
  Discretize(fixed frame)/4(bet) -> choose/4(In4)
  Discretize(fixed frame)/3(Cd) -> choose/3(In3)
  Discretize(fixed frame)/2(Bd) -> choose/2(In2)
  Discretize(fixed frame)/1(Ad) -> choose/1(In1)
  Constant5/1 -> Discretize(fixed frame)/2(be)
  Constant4/1 -> Discretize(fixed frame)/Enable
  [phi] -> Bus Creator/2
  Constant3/1 -> Sum4/1
  u1/1 -> Sum4/2
  [rot_frame] -> Discretize (rotor Frame)/Enable
  Sum4/1 -> [rot_frame]
  [Ic] -> Simulink-PS Converter2/1
  [Ib] -> Simulink-PS Converter1/1
  [Ia] -> Simulink-PS Converter/1
  PS-Simulink Converter2/1 -> [Vc]
  PS-Simulink Converter1/1 -> [Vb]
  PS-Simulink Converter/1 -> [Va]
  Mux/1 -> [Vnode]
  Demux/3 -> [Ic]
  Demux/2 -> [Ib]
  Demux/1 -> [Ia]
  [Vb] -> Mux/2
  [Vc] -> Mux/3
  [Ihist] -> Gain/1
  Gain/1 -> Demux/1
  [Va] -> Mux/1
  Product2/1 -> [omega_flux]
  [phi] -> 1 step prediction+2step averaging/1(In1)
  [omega_flux] -> MATE/7(u_speedterm)
  Mat Function2/1 -> Product5/1
  Constant2/1 -> Discretize (rotor Frame)/4(be)
  [Vnode] -> Unit Delay/1
  [IM2_Tpark] -> Matrix Concatenate1/1
  Mat Function1/1 -> Matrix Concatenate1/2
  rotorzeros/1 -> Mat Function1/1
  Product5/1 -> Discretize (rotor Frame)/3(Cc), Product1/1, Discretize(fixed frame)/1(Cc)
  [IM2_invLdq] -> Product5/2  "Linv"
  Unit Delay/1 -> MATE/4(u)
  Bus Creator/1 -> meas/1
  MATE/3(phi) -> [phi]  "flux d-q stator d-q rotor (Wb)"
  Product1/1 -> Bus Creator/1  "Iabc_stator (A)"
  Matrix Concatenate1/1 -> Discretize (rotor Frame)/2(Bc), Mat Function2/1
  [IM2_Adq] -> Discretize (rotor Frame)/1(Ac)
  [IM2_invLdq] -> Product4/1
  Product4/1 -> Gain9/1
  Gain9/1 -> Mux3/1  "I_dq"
  Gain8/1 -> Mux3/2  "phi_dq"
  Mux3/1 -> Selector5/1, Selector4/1
  Product7/1 -> Sum1/1
  Product9/1 -> Sum1/2
  Selector5/1 -> Product9/1
  Selector4/1 -> Product7/1
  Sum1/1 -> pole pair3/1
  pole pair3/1 -> Bus Creator/3  "Electric torque (Nm)"
  MATE/1(Y) -> Terminator/1
  MATE/2(Ihist) -> [Ihist]
  1 step prediction+2step averaging/1(Out1) -> Product2/2
  [phi] -> Product4/2, Gain8/1
  [phi] -> Product1/2
  Discrete-Time Integrator/1 -> dq_rotortransform/1(angle)  "theta_elect (rad)"
  Matrice/1(Adq) -> [IM2_Adq]
  Matrice/2(invLdq) -> [IM2_invLdq]
  "   w_mec"/1 -> pole pair1/1
  pole pair1/1 -> Discrete-Time Integrator/1, Matrice/1(we)  "w_elect"
  Matrice/3(speed term) -> Product2/1
  Constant1/1 -> Matrice/2(park)
  dq_rotortransform/1(Trotor) -> Switch/1
  Switch/1 -> [IM2_Tpark]
  connections:
  Controlled Current Source1/RConn1 -- Simulink-PS Converter2/RConn1
  Controlled Current Source/RConn1 -- Simulink-PS Converter1/RConn1
  Simulink-PS Converter/RConn1 -- Controlled Current Source2/RConn1
  Voltage Sensor1/RConn1 -- PS-Simulink Converter2/LConn1
  PS-Simulink Converter1/LConn1 -- Voltage Sensor/RConn1
  PS-Simulink Converter/LConn1 -- Voltage Sensor2/RConn1
  Electrical Reference7/LConn1 -- Resistor2/RConn1
  Electrical Reference6/LConn1 -- Controlled Current Source2/RConn2
  Electrical Reference8/LConn1 -- Voltage Sensor2/RConn2
  Phase Splitter/RConn1 -- Voltage Sensor2/LConn1 -- Resistor2/LConn1 -- Resistor3/LConn1 -- Resistor5/LConn1 -- Controlled Current Source2/LConn1
  Electrical Reference4/LConn1 -- Resistor1/RConn1
  Electrical Reference3/LConn1 -- Controlled Current Source1/RConn2
  Electrical Reference5/LConn1 -- Voltage Sensor1/RConn2
  Resistor1/LConn1 -- Resistor4/RConn1 -- Resistor5/RConn1 -- Phase Splitter/RConn3 -- Voltage Sensor1/LConn1 -- Controlled Current Source1/LConn1
  Electrical Reference2/LConn1 -- Voltage Sensor/RConn2
  Electrical Reference1/LConn1 -- Resistor/RConn1
  Resistor/LConn1 -- Resistor3/RConn1 -- Resistor4/LConn1 -- Phase Splitter/RConn2 -- Voltage Sensor/LConn1 -- Controlled Current Source/LConn1
  Electrical Reference/LConn1 -- Controlled Current Source/RConn2
  "   abc"/RConn1 -- Phase Splitter/LConn1

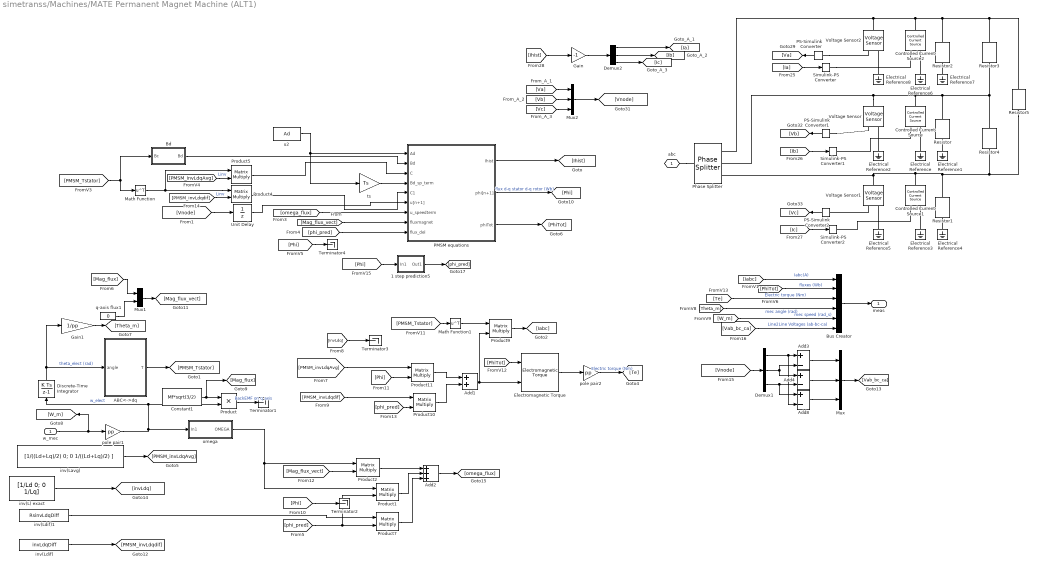
== system simetranss/Machines/MATE Permanent Magnet Machine (ALT1) ==
  "   w_mec" : Inport
  1 step prediction5 : Subsystem
  ABC<->dq : Subsystem
  Add1 : Sum
  Add2 : Sum  Inputs=+++
  Add3 : Sum  Inputs=+-
  Add4 : Sum  Inputs=+-
  Add8 : Sum  Inputs=+-
  Bd : Subsystem
  Bus Creator : BusCreator  Inputs=6
  Constant1 : Constant  Value=Mf*sqrt(3/2)
  Controlled Current Source : fl_lib/Electrical/Electrical Sources/Controlled Current Source
  Controlled Current Source1 : fl_lib/Electrical/Electrical Sources/Controlled Current Source
  Controlled Current Source2 : fl_lib/Electrical/Electrical Sources/Controlled Current Source
  Demux1 : Demux  Outputs=[1 1 1]
  Demux2 : Demux  Outputs=3
      settings: DisplayOption=none
  Discrete-Time Integrator : DiscreteIntegrator  InitialCondition=pp*AngInit/180*pi  SampleTime=Ts  ICPrevOutput=DiscIntNeverNeededParam  ICPrevScaledInput=DiscIntNeverNeededParam
  Electrical Reference{,1..8} (9 alike) : fl_lib/Electrical/Electrical Elements/Electrical Reference
  Electromagnetic Torque : artemis/SSN/SSN rotating machines/SSN Synchronous Machine/Electromagnetic Torque  SystemSampleTime=-1  VariantActivationTime=update diagram  AllowFlexibleInterface=on  Latency=0  AutoFrameSizeCalculation=off
      settings: SourceProductName=Artemis
  Gain : Gain  Gain=-1
  Gain1 : Gain  Gain=1/pp
  Math Function : Math  Operator=transpose  SignedPower=on
  Math Function1 : Math  Operator=transpose  SignedPower=on
  Mux : Mux  Inputs=3
  Mux1 : Mux  Inputs=2
  Mux2 : Mux  Inputs=3
  PMSM equations : Subsystem
  PS-Simulink Converter : nesl_utility/PS-Simulink Converter  PhysicalDomain=network_engine_domain  SubClassName=ps_output  LeftPortType=input  RightPortType=output  PseudoPeriodic=off  Frequencies=[]  VectorFormat=inherit  Unit=inherit  AffineConversion=off
  PS-Simulink Converter1 : nesl_utility/PS-Simulink Converter  PhysicalDomain=network_engine_domain  SubClassName=ps_output  LeftPortType=input  RightPortType=output  PseudoPeriodic=off  Frequencies=[]  VectorFormat=inherit  Unit=inherit  AffineConversion=off
  PS-Simulink Converter2 : nesl_utility/PS-Simulink Converter  PhysicalDomain=network_engine_domain  SubClassName=ps_output  LeftPortType=input  RightPortType=output  PseudoPeriodic=off  Frequencies=[]  VectorFormat=inherit  Unit=inherit  AffineConversion=off
  Phase Splitter : ee_lib/Connectors & References/Phase Splitter
  Product : Product  RndMeth=Zero
  Product{1..2,4..5,7,9..11} (8 alike) : Product  Multiplication=Matrix(*)  SaturateOnIntegerOverflow=on  OutDataTypeStr=Inherit: Same as first input
  Resistor : fl_lib/Electrical/Electrical Elements/Resistor  R=ResistanceM(2,2) Ohm  i_specify=off  i_priority=None  i=0 A  i_nominal_specify=off  i_nominal_value=1  i_nominal_unit=A  v_specify=off  v_priority=None  v=0 V  v_nominal_specify=off  v_nominal_value=1  v_nominal_unit=V
  Resistor1 : fl_lib/Electrical/Electrical Elements/Resistor  R=ResistanceM(3,3) Ohm  i_specify=off  i_priority=None  i=0 A  i_nominal_specify=off  i_nominal_value=1  i_nominal_unit=A  v_specify=off  v_priority=None  v=0 V  v_nominal_specify=off  v_nominal_value=1  v_nominal_unit=V
  Resistor2 : fl_lib/Electrical/Electrical Elements/Resistor  R=ResistanceM(1,1) Ohm  i_specify=off  i_priority=None  i=0 A  i_nominal_specify=off  i_nominal_value=1  i_nominal_unit=A  v_specify=off  v_priority=None  v=0 V  v_nominal_specify=off  v_nominal_value=1  v_nominal_unit=V
  Resistor3 : fl_lib/Electrical/Electrical Elements/Resistor  R=ResistanceM(1,2) Ohm  i_specify=off  i_priority=None  i=0 A  i_nominal_specify=off  i_nominal_value=1  i_nominal_unit=A  v_specify=off  v_priority=None  v=0 V  v_nominal_specify=off  v_nominal_value=1  v_nominal_unit=V
  Resistor4 : fl_lib/Electrical/Electrical Elements/Resistor  R=ResistanceM(2,3) Ohm  i_specify=off  i_priority=None  i=0 A  i_nominal_specify=off  i_nominal_value=1  i_nominal_unit=A  v_specify=off  v_priority=None  v=0 V  v_nominal_specify=off  v_nominal_value=1  v_nominal_unit=V
  Resistor5 : fl_lib/Electrical/Electrical Elements/Resistor  R=ResistanceM(1,3) Ohm  i_specify=off  i_priority=None  i=0 A  i_nominal_specify=off  i_nominal_value=1  i_nominal_unit=A  v_specify=off  v_priority=None  v=0 V  v_nominal_specify=off  v_nominal_value=1  v_nominal_unit=V
  Simulink-PS Converter : nesl_utility/Simulink-PS Converter  PhysicalDomain=network_engine_domain  SubClassName=ps_input  LeftPortType=input  RightPortType=output  PseudoPeriodic=off  Frequencies=[]  NoiseDistribution=none  NoiseParameters=[]  Unit=1  AffineConversion=off  FilteringAndDerivatives=provide  SimscapeFilterOrder=1  InputFilterTimeConstant=0.001  UdotUserProvided=0
  Simulink-PS Converter1 : nesl_utility/Simulink-PS Converter  PhysicalDomain=network_engine_domain  SubClassName=ps_input  LeftPortType=input  RightPortType=output  PseudoPeriodic=off  Frequencies=[]  NoiseDistribution=none  NoiseParameters=[]  Unit=1  AffineConversion=off  FilteringAndDerivatives=provide  SimscapeFilterOrder=1  InputFilterTimeConstant=0.001  UdotUserProvided=0
  Simulink-PS Converter2 : nesl_utility/Simulink-PS Converter  PhysicalDomain=network_engine_domain  SubClassName=ps_input  LeftPortType=input  RightPortType=output  PseudoPeriodic=off  Frequencies=[]  NoiseDistribution=none  NoiseParameters=[]  Unit=1  AffineConversion=off  FilteringAndDerivatives=provide  SimscapeFilterOrder=1  InputFilterTimeConstant=0.001  UdotUserProvided=0
  Terminator{1..4} (4 alike) : Terminator
  Unit Delay : UnitDelay  SampleTime=Ts  HasFrameUpgradeWarning=on
  Voltage Sensor : fl_lib/Electrical/Electrical Sensors/Voltage Sensor
  Voltage Sensor1 : fl_lib/Electrical/Electrical Sensors/Voltage Sensor
  Voltage Sensor2 : fl_lib/Electrical/Electrical Sensors/Voltage Sensor
  inv(L) exact : Constant  Value=[1/Ld 0; 0 1/Lq]
  inv(Lavg) : Constant  Value=[1/((Ld+Lq)/2) 0; 0 1/((Ld+Lq)/2) ]
  inv(Ldif) : Constant  Value=invLdqDiff
  inv(Ldif)1 : Constant  Value=RsinvLdqDiff
  omega : Subsystem
  pole pair1 : Gain  Gain=pp
  pole pair2 : Gain  Gain=pp
  q-axis flux1 : Constant  Value=0
  ts : Gain  Gain=Ts  SaturateOnIntegerOverflow=on  OutDataTypeStr=Inherit: Same as input  ParamDataTypeStr=Inherit: Same as input
  u2 : Constant  Value=Ad
  "   abc" : PMIOPort  Side=Left
  meas : Outport  VectorParamsAs1DForOutWhenUnconnected=off
  wires:
  omega/1(OMEGA) -> Product2/1, Product1/1
  ts/1 -> PMSM equations/4(Bd_sp_term)
  u2/1 -> PMSM equations/1(Ad), ts/1
  [Ihist] -> Gain/1
  Demux2/3 -> [Ic]
  [Ib] -> Simulink-PS Converter1/1
  PS-Simulink Converter/1 -> [Va]
  [Ic] -> Simulink-PS Converter2/1
  PS-Simulink Converter1/1 -> [Vb]
  Demux2/2 -> [Ib]
  [Va] -> Mux2/1
  PS-Simulink Converter2/1 -> [Vc]
  [Vb] -> Mux2/2
  [Ia] -> Simulink-PS Converter/1
  Mux2/1 -> [Vnode]
  Gain/1 -> Demux2/1
  [Vc] -> Mux2/3
  Demux2/1 -> [Ia]
  [Vab_bc_ca] -> Bus Creator/6  "Line2Line Voltages (ab-bc-ca)"
  [Vnode] -> Demux1/1
  Demux1/1 -> Add8/2, Add3/1
  Add3/1 -> Mux/1
  Add4/1 -> Mux/2
  Demux1/2 -> Add3/2, Add4/1
  Demux1/3 -> Add8/1, Add4/2
  Mux/1 -> [Vab_bc_ca]
  Add8/1 -> Mux/3
  PMSM equations/1(Ihist) -> [Ihist]
  [Theta_m] -> Bus Creator/4  "mec angle (rad)"
  [W_m] -> Bus Creator/5  "mec speed (rad_s)"
  Gain1/1 -> [Theta_m]
  [PhiTot] -> Bus Creator/2  "fluxes (Wb)"
  [Iabc] -> Bus Creator/1  "Iabc(A)"
  Discrete-Time Integrator/1 -> Gain1/1, ABC<->dq/1(angle)  "theta_elect (rad)"
  [Vnode] -> Unit Delay/1
  [PMSM_Tstator] -> Bd/1(Bc), Math Function/1
  Math Function/1 -> Product5/1, Product4/1
  [PMSM_invLdqAvg] -> Product5/2  "Linv"
  pole pair1/1 -> omega/1(In1), Product/2, Discrete-Time Integrator/1  "w_elect"
  "   w_mec"/1 -> [W_m], pole pair1/1
  inv(Lavg)/1 -> [PMSM_invLdqAvg]
  Bus Creator/1 -> meas/1
  PMSM equations/2(phi[n+1]) -> [Phi]  "flux d-q stator d-q rotor (Wb)"
  Bd/1(Bd) -> PMSM equations/2(Bd)
  Product5/1 -> PMSM equations/3(C)
  ABC<->dq/1(T) -> [PMSM_Tstator]
  Constant1/1 -> [Mag_flux], Product/1
  Product/1 -> Terminator1/1  "BackEMF on q axis"
  Unit Delay/1 -> PMSM equations/6(u[n+1])
  [omega_flux] -> PMSM equations/7(u_speedterm)
  PMSM equations/3(phiTot) -> [PhiTot]
  [PhiTot] -> Electromagnetic Torque/1
  [Te] -> Bus Creator/3  "Electric torque (Nm)"
  pole pair2/1 -> [Te]  "Electric torque (Nm)"
  Product2/1 -> Add2/1
  inv(Ldif)1/1 -> Product7/1
  [Mag_flux] -> Mux1/1
  q-axis flux1/1 -> Mux1/2
  Mux1/1 -> [Mag_flux_vect]
  [Mag_flux_vect] -> PMSM equations/8(fluxmagnet)
  Electromagnetic Torque/1 -> pole pair2/1
  inv(Ldif)/1 -> [PMSM_invLdqdif]
  [Mag_flux_vect] -> Product2/2
  Product9/1 -> [Iabc]
  [invLdq] -> Terminator3/1
  Add1/1 -> Product9/2, Electromagnetic Torque/2
  inv(L) exact/1 -> [invLdq]
  Add2/1 -> [omega_flux]
  [PMSM_Tstator] -> Math Function1/1
  Math Function1/1 -> Product9/1
  [Phi] -> 1 step prediction5/1(In1)
  1 step prediction5/1(Out1) -> [phi_pred]
  Product7/1 -> Add2/3
  Product1/1 -> Add2/2
  [PMSM_invLdqdif] -> Product4/2  "Linv"
  Product4/1 -> PMSM equations/5(C1)
  [phi_pred] -> PMSM equations/9(flux_del)
  [phi_pred] -> Product1/2, Product7/2
  [Phi] -> Product11/2
  [PMSM_invLdqAvg] -> Product11/1
  [PMSM_invLdqdif] -> Product10/1
  [phi_pred] -> Product10/2
  Product11/1 -> Add1/1
  Product10/1 -> Add1/2
  [Phi] -> Terminator2/1
  [Phi] -> Terminator4/1
  connections:
  PS-Simulink Converter1/LConn1 -- Voltage Sensor/RConn1
  Electrical Reference/LConn1 -- Controlled Current Source/RConn2
  Electrical Reference8/LConn1 -- Voltage Sensor2/RConn2
  Electrical Reference4/LConn1 -- Resistor1/RConn1
  Electrical Reference1/LConn1 -- Resistor/RConn1
  PS-Simulink Converter/LConn1 -- Voltage Sensor2/RConn1
  Electrical Reference6/LConn1 -- Controlled Current Source2/RConn2
  "   abc"/RConn1 -- Phase Splitter/LConn1
  Controlled Current Source1/RConn1 -- Simulink-PS Converter2/RConn1
  Controlled Current Source/RConn1 -- Simulink-PS Converter1/RConn1
  Electrical Reference5/LConn1 -- Voltage Sensor1/RConn2
  Simulink-PS Converter/RConn1 -- Controlled Current Source2/RConn1
  Electrical Reference2/LConn1 -- Voltage Sensor/RConn2
  Electrical Reference7/LConn1 -- Resistor2/RConn1
  Voltage Sensor1/RConn1 -- PS-Simulink Converter2/LConn1
  Electrical Reference3/LConn1 -- Controlled Current Source1/RConn2
  Controlled Current Source2/LConn1 -- Resistor2/LConn1 -- Resistor5/LConn1 -- Resistor3/LConn1 -- Voltage Sensor2/LConn1 -- Phase Splitter/RConn1
  Voltage Sensor/LConn1 -- Phase Splitter/RConn2 -- Controlled Current Source/LConn1 -- Resistor/LConn1 -- Resistor3/RConn1 -- Resistor4/LConn1
  Resistor4/RConn1 -- Resistor1/LConn1 -- Voltage Sensor1/LConn1 -- Phase Splitter/RConn3 -- Controlled Current Source1/LConn1 -- Resistor5/RConn1
